simulink model "DACwithSlewRate"  (R2024b)
settings: Solver=VariableStepAuto  StartTime=0.0  StopTime=10.0  RelTol=1e-3
values from neighbouring files (symbols this model uses):
  sr = 1e4    (= 10000)    [main.m]
  Ts = 1/Fs    (= 1e-06)    [getControlMHOQ_RL.m]    (also in main.m; run_linmethods.m; scrapefile.m = 0.0001)
settings Model: Creator=bikashadhikari  LastModifiedBy=bikashadhikari

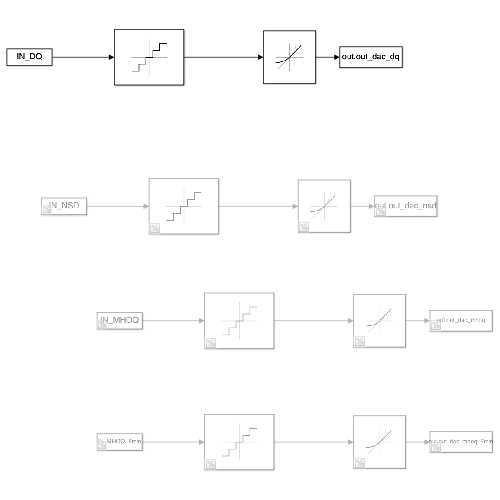
[thumbnail: Simulink's stored preview of the top-level diagram]
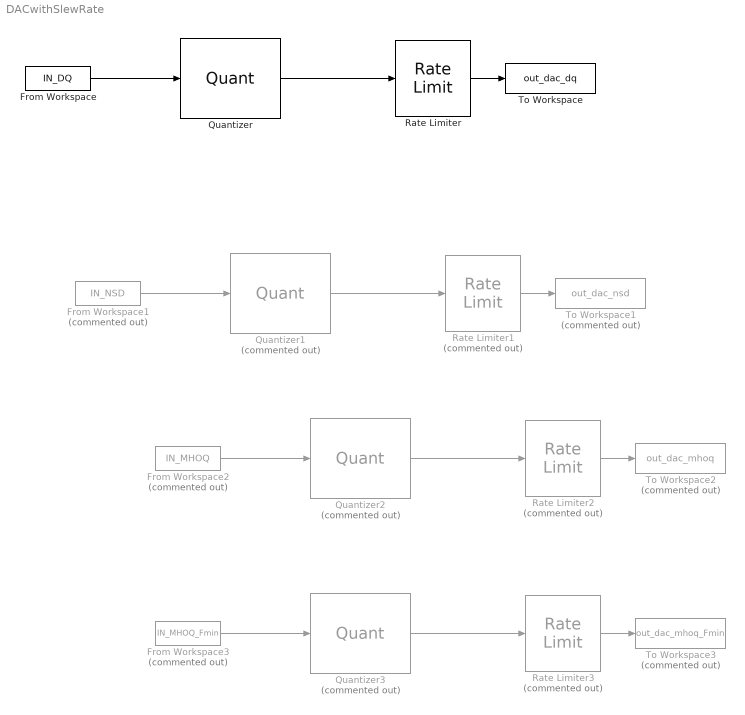
== system DACwithSlewRate ==
  From Workspace : FromWorkspace  VariableName=IN_DQ  SampleTime=Ts
  From Workspace1 : FromWorkspace  Commented=on  VariableName=IN_NSD  SampleTime=Ts
  From Workspace2 : FromWorkspace  Commented=on  VariableName=IN_MHOQ  SampleTime=Ts
  From Workspace3 : FromWorkspace  Commented=on  VariableName=IN_MHOQ_Fmin  SampleTime=Ts
  Quantizer : Quantizer  QuantizationInterval=Qstep
  Quantizer1 : Quantizer  Commented=on  QuantizationInterval=Qstep
  Quantizer2 : Quantizer  Commented=on  QuantizationInterval=Qstep
  Quantizer3 : Quantizer  Commented=on  QuantizationInterval=Qstep
  Rate Limiter : RateLimiter  RisingSlewLimit=sr  FallingSlewLimit=-sr  SampleTimeMode=inherited
  Rate Limiter1 : RateLimiter  Commented=on  RisingSlewLimit=sr  FallingSlewLimit=-sr  SampleTimeMode=inherited
  Rate Limiter2 : RateLimiter  Commented=on  RisingSlewLimit=sr  FallingSlewLimit=-sr  SampleTimeMode=inherited
  Rate Limiter3 : RateLimiter  Commented=on  RisingSlewLimit=sr  FallingSlewLimit=-sr  SampleTimeMode=inherited
  To Workspace : ToWorkspace  VariableName=out_dac_dq  SaveFormat=Timeseries  SampleTime=Ts
  To Workspace1 : ToWorkspace  Commented=on  VariableName=out_dac_nsd  SaveFormat=Timeseries  SampleTime=Ts
  To Workspace2 : ToWorkspace  Commented=on  VariableName=out_dac_mhoq  SaveFormat=Timeseries  SampleTime=Ts
  To Workspace3 : ToWorkspace  Commented=on  VariableName=out_dac_mhoq_Fmin  SaveFormat=Timeseries  SampleTime=Ts
  wires:
  Rate Limiter/1 -> To Workspace/1
  Quantizer/1 -> Rate Limiter/1
  From Workspace/1 -> Quantizer/1
  Quantizer1/1 -> Rate Limiter1/1
  From Workspace1/1 -> Quantizer1/1
  Rate Limiter1/1 -> To Workspace1/1
  Quantizer2/1 -> Rate Limiter2/1
  From Workspace2/1 -> Quantizer2/1
  Rate Limiter2/1 -> To Workspace2/1
  Quantizer3/1 -> Rate Limiter3/1
  Rate Limiter3/1 -> To Workspace3/1
  From Workspace3/1 -> Quantizer3/1
